simulink model "ZT_VehCtrl_18B"  (R2018b)
settings: Solver=FixedStepAuto  StartTime=0.0  StopTime=inf  FixedStep=0.005  RelTol=1e-3
InitFcn:
  | mbd_mpc_consistency_checks(bdroot(gcs));
undefined symbols (not defined in the file): ANG_DEAD, BMS_NormalPwr, BrkPrsByBrkPct_TB_X, BrkPrsByBrkPct_TB_Y, DELAY_DISCHARGE, DELAY_RCUOFF, DRV_BACKWARD, DRV_BRAKE, DRV_FORWARD, DRV_NEUTRAL, DRV_PARK, DRV_UNPARK, DRV_ZEROTURN, EPB_LOCK, EPB_UNLOCK, ExtraLoadPwr, FanOff, fifo_0_vect, fifo_1_vect, HiFanReq, HV_finished, HV_No_Active, HV_POWER_OFF, HV_POWER_ON, HVDown, HVON, KaTLS_v_DrgUp_X_VehSpd, KeFTM_s_Way1OffDlyTime, KeFTM_TK_Way1CoolLv2OffBatTemp, KeFTM_TK_Way1CoolLv2OffMtrTemp, KeFTM_TK_Way1CoolLv2OnBatTemp, KeFTM_TK_Way1CoolLv2OnMtrTemp, KeFTM_TK_Way1CoolLv3OffBatTemp, KeFTM_TK_Way1CoolLv3OffMtrTemp, KeFTM_TK_Way1CoolLv3OnBatTemp, KeFTM_TK_Way1CoolLv3OnMtrTemp, KeFTM_TK_Way1CoolLv4OffBatTemp, KeFTM_TK_Way1CoolLv4OffMtrTemp, KeFTM_TK_Way1CoolLv4OnBatTemp, KeFTM_TK_Way1CoolLv4OnMtrTemp, Kp1, Kp2, LowFanReq, LQFP, MtrPwrFactor_RCU, MtrPwrHighToMidThd, MtrPwrLowToMidThd, MtrPwrMidToHighThd, MtrPwrMidToLowThd, MtrTrqMax, PCT_DEAD, Precharge, PTO_1000, PTO_540, pts1_fifo_0_vect, pts1_fifo_1_vect, pts2_fifo_0_vect, pts2_fifo_1_vect, pts3_fifo_0_vect, pts3_fifo_1_vect ... (+24)
libraries: mbd_mpc574x_ec_toolbox x124, canmsglib x72, simulink x57
(part 2 of 11)

== system ZT_VehCtrl_18B/Initialization & SPI timer1 ==
  note: 由于SPI0用了两个片选，SPI3只用了一个片选（没算EEPROM）。
      | 因此直接用方波就可以了。
      | 如果增加SPI控制，建议使用StateFlow构造激活函数。
      | 由于模版使用的0.01s的仿真步长，这里构造周期为0.02s,占空比为0.5的方波。
  note: SPI3
  note: SPI0
  CS1 LS : Subsystem
  CS2 CANB : Subsystem
  CS3 LS : Subsystem
  CS5 LS : Subsystem
  Chart : Stateflow chart  TreatAsAtomicUnit=on
  Chart1 : Stateflow chart  TreatAsAtomicUnit=on
  Chart2 : Stateflow chart  TreatAsAtomicUnit=on
  Compare To Constant : simulink/Logic and Bit Operations/Compare To Constant  relop===  const=9  OutDataTypeStr=boolean
  Compare To Constant1 : simulink/Logic and Bit Operations/Compare To Constant  relop===  const=9  OutDataTypeStr=boolean
  Constant : Constant
  Data Store Read : DataStoreRead  DataStoreName=VCU_Mode
  Data Store Read1 : DataStoreRead  DataStoreName=ResetFlg
  Data Store Read2 : DataStoreRead  DataStoreName=Init_flg_SPI
  Data Store Write : DataStoreWrite  DataStoreName=VCU_Mode
  Data Store Write2 : DataStoreWrite  DataStoreName=SPI0_CS
  Data Store Write3 : DataStoreWrite  DataStoreName=SPI3_CS
  Data Store Write4 : DataStoreWrite  DataStoreName=Init_flg_SPI
  Data Type Conversion{,1..3} (4 alike) : DataTypeConversion
  If : If  IfExpression=u1 == 1  ShowElse=off
  If1 : If  IfExpression=u1 == 1  ShowElse=off
  If2 : If  IfExpression=u1 == 2  ShowElse=off
  If3 : If  IfExpression=u1 == 2  ShowElse=off
  Logical Operator : Logic  AllPortsSameDT=off  OutDataTypeStr=boolean
  Pulse Generator : DiscretePulseGenerator  PulseType=Time based  Period=0.01  PulseWidth=50
  wires:
  If/1 -> CS2 CANB/Action
  Chart/1(Flg) -> Data Type Conversion3/1
  Data Store Read2/1 -> Chart/2(InitFlg)
  If1/1 -> CS1 LS/Action
  Chart2/1(Flg) -> If3/1, [SPI3_flg], If/1
  Data Store Read/1 -> Chart2/1(VcuMode), Chart1/1(VcuMode)
  If2/1 -> CS5 LS/Action
  [SPI0_flg] -> Compare To Constant/1
  [SPI3_flg] -> Compare To Constant1/1
  Compare To Constant/1 -> Logical Operator/1
  Compare To Constant1/1 -> Logical Operator/2
  Logical Operator/1 -> Data Type Conversion2/1
  If3/1 -> CS3 LS/Action
  Pulse Generator/1 -> Data Type Conversion/1
  Constant/1 -> Data Type Conversion1/1
  Data Type Conversion/1 -> Data Store Write2/1
  Data Type Conversion1/1 -> Data Store Write3/1
  Data Type Conversion2/1 -> Data Store Write4/1
  Data Type Conversion3/1 -> Data Store Write/1
  Chart1/1(Flg) -> If1/1, [SPI0_flg], If2/1
  Data Store Read1/1 -> Chart/1(ResetFlg)

== system ZT_VehCtrl_18B/Power Managment ==
  PowerMode : Inport
  Data Type Conversion : DataTypeConversion
  HS1 : mbd_mpc574x_ec_toolbox/GPIO Blocks/Digital_Output  Priority=1  gpio_pin=PTF6: [SIUL2_GPIO86 | General Purpose IO PF[6]]  gpio_drive_strength=Disabled
  HS4 : mbd_mpc574x_ec_toolbox/GPIO Blocks/Digital_Output  Priority=1  gpio_pin=PTA13: [SIUL2_GPIO13 | General Purpose IO PA[13]]  gpio_drive_strength=Disabled
  wires:
  PowerMode/1 -> Data Type Conversion/1
  Data Type Conversion/1 -> HS4/1, HS1/1

== system ZT_VehCtrl_18B/SPI_EEPROM ==
  Data Store Memory : DataStoreMemory  DataStoreName=A_write  ReadBeforeWriteMsg=warning  WriteAfterWriteMsg=warning  WriteAfterReadMsg=warning  ShowAdditionalParam=off  OutDataTypeStr=single
      settings: RTWStateStorageClass=ExportedGlobal
  Data Store Memory10 : DataStoreMemory  DataStoreName=A_read  ReadBeforeWriteMsg=warning  WriteAfterWriteMsg=warning  WriteAfterReadMsg=warning  ShowAdditionalParam=off  OutDataTypeStr=single
      settings: RTWStateStorageClass=ExportedGlobal
  Data Store Memory18 : DataStoreMemory  DataStoreName=SPI0_CTRL0  ReadBeforeWriteMsg=warning  WriteAfterWriteMsg=warning  WriteAfterReadMsg=warning  ShowAdditionalParam=off  OutDataTypeStr=uint8
      settings: RTWStateStorageClass=ExportedGlobal
  Data Store Read : DataStoreRead  DataStoreName=SPI0_CTRL0
  SPI_read : Subsystem  TreatAsAtomicUnit=on
  SPI_write : Subsystem  TreatAsAtomicUnit=on
  Switch Case : SwitchCase  CaseConditions={1,2}  ShowDefaultCase=off
  wires:
  Data Store Read/1 -> Switch Case/1
  Switch Case/2 -> SPI_write/Action
  Switch Case/1 -> SPI_read/Action

== system ZT_VehCtrl_18B/SigIn ==
  note: CAN0
  note: HardWareSignalIn
  note: CAN1
  AI : Subsystem
  "CAN0 " : Subsystem  TreatAsAtomicUnit=on
      settings: RTWSystemCode=Nonreusable function
  CAN0_Rx_500 : mbd_mpc574x_ec_toolbox/Communication Blocks/CAN Blocks/FCAN_Isr  can_instance=0  can_event=Rx Complete
      settings: SourceProductName=NXP Model-Based Design Toolbox for MPC57xx MCUs
  CAN1 : Subsystem  TreatAsAtomicUnit=on
      settings: RTWSystemCode=Nonreusable function
  CAN1_Rx_500 : mbd_mpc574x_ec_toolbox/Communication Blocks/CAN Blocks/FCAN_Isr  can_instance=1  can_event=Rx Complete
      settings: SourceProductName=NXP Model-Based Design Toolbox for MPC57xx MCUs
  DI : Subsystem
  PWM : Subsystem
  Terminator{,3..5,8} (5 alike) : Terminator
  MCU_FL : Outport  VectorParamsAs1DForOutWhenUnconnected=on
  MCU_FR : Outport  Port=2  VectorParamsAs1DForOutWhenUnconnected=on
  MCU_RL : Outport  Port=3  VectorParamsAs1DForOutWhenUnconnected=on
  MCU_RR : Outport  Port=4  VectorParamsAs1DForOutWhenUnconnected=on
  MCU1 : Outport  Port=5  VectorParamsAs1DForOutWhenUnconnected=on
  MCU2 : Outport  Port=6  VectorParamsAs1DForOutWhenUnconnected=on
  HVC : Outport  Port=7  VectorParamsAs1DForOutWhenUnconnected=on
  ACU : Outport  Port=8  VectorParamsAs1DForOutWhenUnconnected=on
  PDU : Outport  Port=9  VectorParamsAs1DForOutWhenUnconnected=on
  TWV : Outport  Port=10  VectorParamsAs1DForOutWhenUnconnected=on
  TMS : Outport  Port=11  VectorParamsAs1DForOutWhenUnconnected=on
  ISG : Outport  Port=12  VectorParamsAs1DForOutWhenUnconnected=on
  wires:
  CAN1_Rx_500/2 -> Terminator4/1
  CAN1_Rx_500/6 -> CAN1/4(timestamp)
  CAN1_Rx_500/4 -> CAN1/2(Data)
  CAN1_Rx_500/3 -> CAN1/1(ID)
  CAN1_Rx_500/5 -> CAN1/3(length)
  CAN0_Rx_500/5 -> "CAN0 "/3(length)
  CAN0_Rx_500/3 -> "CAN0 "/1(ID)
  CAN0_Rx_500/4 -> "CAN0 "/2(Data)
  CAN0_Rx_500/6 -> "CAN0 "/4(timestamp)
  CAN0_Rx_500/1 -> "CAN0 "/Trigger
  CAN0_Rx_500/2 -> Terminator8/1
  "CAN0 "/1(BMS) -> MCU_FL/1
  "CAN0 "/2(OBC) -> MCU_FR/1
  "CAN0 "/4("BRS ") -> MCU_RR/1
  "CAN0 "/3(TMS) -> MCU_RL/1
  CAN1_Rx_500/1 -> CAN1/Trigger
  PWM/1(PWMIn) -> Terminator/1
  DI/1(DI) -> Terminator3/1
  AI/1(AI) -> Terminator5/1
  CAN1/1(MCU1) -> MCU1/1
  CAN1/3(HVC) -> HVC/1
  CAN1/7(TMS) -> TMS/1
  CAN1/8("ISG ") -> ISG/1
  CAN1/6(TWV) -> TWV/1
  CAN1/5(PDU) -> PDU/1
  CAN1/4(ACU) -> ACU/1
  CAN1/2(MCU2) -> MCU2/1

== system ZT_VehCtrl_18B/SigOut ==
  note: 10ms
  note: 500ms
  note: 100ms
  note: 200ms
  BMS_OUT : Inport
  ICU : Inport  Port=2
  TMS_OUT1 : Inport  Port=3
  BRS_OUT : Inport  Port=4
  "DCDC_OUT " : Inport  Port=5
  HVC_OUT : Inport  Port=6
  MCU_OUT : Inport  Port=7
  ACU_OUT : Inport  Port=8
  PDU_OUT : Inport  Port=9
  TM_OUT : Inport  Port=10
  ISG_OUT : Inport  Port=11
  TWV_OUT : Inport  Port=12
  ACU : Subsystem  TreatAsAtomicUnit=on  SystemSampleTime=0.01
  BMS : Subsystem  TreatAsAtomicUnit=on  SystemSampleTime=0.01
  BRS : Subsystem  TreatAsAtomicUnit=on  SystemSampleTime=0.01
  DCDC : Subsystem  TreatAsAtomicUnit=on  SystemSampleTime=0.01
  "GPIO " : Subsystem
  HVC : Subsystem  TreatAsAtomicUnit=on  SystemSampleTime=0.01
  "ICU1 " : Subsystem  TreatAsAtomicUnit=on  SystemSampleTime=0.01
  ICU2 : Subsystem  TreatAsAtomicUnit=on  SystemSampleTime=0.01
  ISG : Subsystem  TreatAsAtomicUnit=on  SystemSampleTime=0.01
  MCU : Subsystem  TreatAsAtomicUnit=on  SystemSampleTime=0.01
  PDU : Subsystem  TreatAsAtomicUnit=on  SystemSampleTime=0.01
  Pulse Generator : DiscretePulseGenerator  PulseType=Time based  Period=0.1  PulseWidth=50
  Pulse Generator1 : DiscretePulseGenerator  PulseType=Time based  Period=0.01  PulseWidth=50
  Pulse Generator2 : DiscretePulseGenerator  PulseType=Time based  Period=0.5  PulseWidth=50
  Pulse Generator6 : DiscretePulseGenerator  PulseType=Time based  Period=0.2  PulseWidth=50
  Rate Transition{,1..4,6..13} (13 alike) : RateTransition
  TM : Subsystem  TreatAsAtomicUnit=on  SystemSampleTime=0.01
  TMS1 : Subsystem  TreatAsAtomicUnit=on  SystemSampleTime=0.01
  TWV : Subsystem  TreatAsAtomicUnit=on  SystemSampleTime=0.01
  wires:
  Pulse Generator2/1 -> ICU2/Trigger
  BMS_OUT/1 -> Rate Transition/1
  Rate Transition/1 -> BMS/1("BMS_OUT ")
  Rate Transition4/1 -> ICU2/1("ICU_OUT ")
  Pulse Generator/1 -> BRS/Trigger, "ICU1 "/Trigger, DCDC/Trigger, HVC/Trigger, TWV/Trigger, PDU/Trigger, ACU/Trigger, BMS/Trigger
  ICU/1 -> Rate Transition4/1, Rate Transition6/1
  Rate Transition6/1 -> "ICU1 "/1("ICU_OUT ")
  TMS_OUT1/1 -> Rate Transition7/1
  Rate Transition7/1 -> TMS1/1("TMS_OUT ")
  Pulse Generator6/1 -> TMS1/Trigger
  BRS_OUT/1 -> Rate Transition8/1
  Rate Transition8/1 -> BRS/1("BRS_OUT ")
  Rate Transition1/1 -> DCDC/1("DCDC_OUT ")
  "DCDC_OUT "/1 -> Rate Transition1/1
  HVC_OUT/1 -> Rate Transition2/1
  Rate Transition2/1 -> HVC/1("HVC_OUT ")
  Rate Transition3/1 -> MCU/1("MCU_OUT ")
  MCU_OUT/1 -> Rate Transition3/1
  Rate Transition9/1 -> ACU/1("ACU_OUT ")
  ACU_OUT/1 -> Rate Transition9/1
  PDU_OUT/1 -> Rate Transition10/1
  Rate Transition10/1 -> PDU/1("PDU_OUT ")
  TM_OUT/1 -> Rate Transition11/1
  Rate Transition11/1 -> TM/1("TM_OUT ")
  Rate Transition12/1 -> ISG/1("ISG_OUT ")
  ISG_OUT/1 -> Rate Transition12/1
  Pulse Generator1/1 -> MCU/Trigger, ISG/Trigger, TM/Trigger
  Rate Transition13/1 -> TWV/1("TWV_OUT ")
  TWV_OUT/1 -> Rate Transition13/1

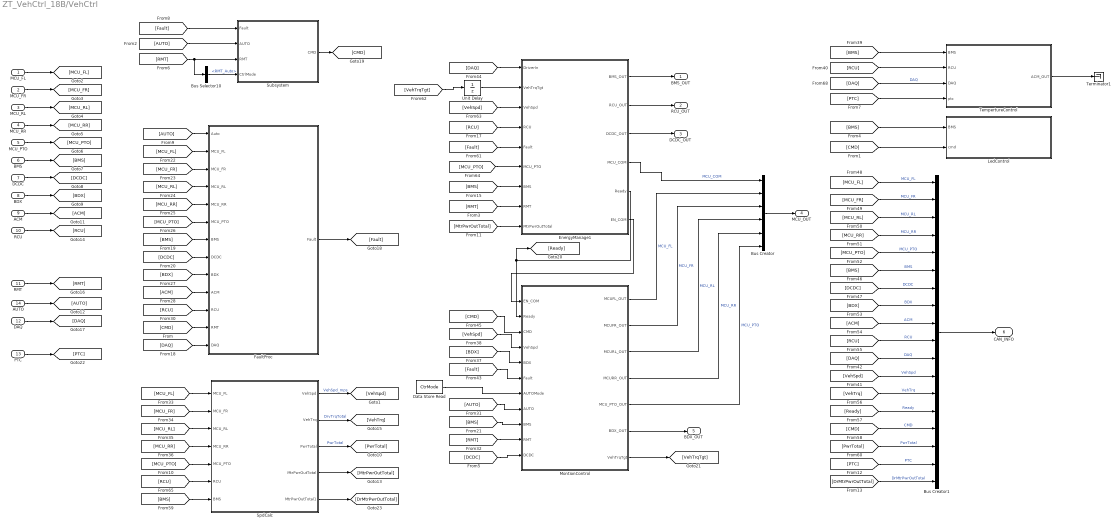
== system ZT_VehCtrl_18B/VehCtrl ==
  MCU_FL : Inport
  MCU_FR : Inport  Port=2
  MCU_RL : Inport  Port=3
  MCU_RR : Inport  Port=4
  MCU_PTO : Inport  Port=5
  BMS : Inport  Port=6
  DCDC : Inport  Port=7
  BDX : Inport  Port=8
  ACM : Inport  Port=9
  RCU : Inport  Port=10
  RMT : Inport  Port=11
  DAQ : Inport  Port=12
  "PTC " : Inport  Port=13
  AUTO : Inport  Port=14
  Bus Creator : BusCreator  Inputs=6
  Bus Creator1 : BusCreator  Inputs=18
  Bus Selector10 : BusSelector  OutputSignals=RMT3.RMT_Auto
  Data Store Read : DataStoreRead  DataStoreName=CtrMode
  EnergyManage1 : Subsystem
  FaultProc : Subsystem
  LedControl : Subsystem
  MontionControl : Subsystem
  SpdCalc : Subsystem
  Subsystem : Subsystem
  TempertureControl : Subsystem
  Terminator1 : Terminator
  Unit Delay : UnitDelay  SampleTime=-1
  BMS_OUT : Outport
  RCU_OUT : Outport  Port=2
  DCDC_OUT : Outport  Port=3
  MCU_OUT : Outport  Port=4
  BDX_OUT : Outport  Port=5
  CAN_INFO : Outport  Port=6
  wires:
  MCU_FL/1 -> [MCU_FL]
  MCU_FR/1 -> [MCU_FR]
  MCU_RR/1 -> [MCU_RR]
  MCU_RL/1 -> [MCU_RL]
  DCDC/1 -> [DCDC]
  BDX/1 -> [BDX]
  BMS/1 -> [BMS]
  MCU_PTO/1 -> [MCU_PTO]
  RMT/1 -> [RMT]
  DAQ/1 -> [DAQ]
  RCU/1 -> [RCU]
  ACM/1 -> [ACM]
  [RCU] -> EnergyManage1/4(RCU)
  [MCU_FL] -> FaultProc/2(MCU_FL)
  [MCU_FR] -> FaultProc/3(MCU_FR)
  [MCU_RL] -> FaultProc/4(MCU_RL)
  [MCU_RR] -> FaultProc/5(MCU_RR)
  [MCU_PTO] -> FaultProc/6(MCU_PTO)
  [BMS] -> FaultProc/7(BMS)
  [DCDC] -> FaultProc/8(DCDC)
  [BDX] -> FaultProc/9(BDX)
  [ACM] -> FaultProc/10(ACM)
  [RCU] -> FaultProc/11(RCU)
  [CMD] -> FaultProc/12(RMT)
  [DAQ] -> FaultProc/13(DAQ)
  [BDX] -> MontionControl/5(BDX)
  [VehSpd] -> MontionControl/4(VehSpd)
  FaultProc/1(Fault) -> [Fault]
  [Fault] -> MontionControl/6(Fault)
  [DAQ] -> EnergyManage1/1(DriverIn)
  [CMD] -> MontionControl/3(CMD)
  [Fault] -> EnergyManage1/5(Fault)
  MontionControl/7(VehTrqTgt) -> [VehTrqTgt]
  [VehTrqTgt] -> Unit Delay/1
  [VehSpd] -> EnergyManage1/3(VehSpd)
  [MCU_PTO] -> EnergyManage1/6(MCU_PTO)
  [BMS] -> EnergyManage1/7(BMS)
  Unit Delay/1 -> EnergyManage1/2(VehTrqTgt)
  EnergyManage1/4(MCU_COM) -> Bus Creator/1  "MCU_COM"
  Bus Creator/1 -> MCU_OUT/1
  EnergyManage1/1(BMS_OUT) -> BMS_OUT/1
  EnergyManage1/2(RCU_OUT) -> RCU_OUT/1
  EnergyManage1/3(DCDC_OUT) -> DCDC_OUT/1
  MontionControl/1(MCUFL_OUT) -> Bus Creator/2  "MCU_FL"
  MontionControl/2(MCUFR_OUT) -> Bus Creator/3  "MCU_FR"
  MontionControl/3(MCURL_OUT) -> Bus Creator/4  "MCU_RL"
  MontionControl/4(MCURR_OUT) -> Bus Creator/5  "MCU_RR"
  MontionControl/5(MCU_PTO_OUT) -> Bus Creator/6  "MCU_PTO"
  MontionControl/6(BDX_OUT) -> BDX_OUT/1
  "PTC "/1 -> [PTC]
  AUTO/1 -> [AUTO]
  [AUTO] -> Subsystem/2(AUTO)
  Subsystem/1(CMD) -> [CMD]
  Data Store Read/1 -> MontionControl/7(AUTOMode)
  [AUTO] -> MontionControl/8(AUTO)
  Bus Selector10/1 -> Subsystem/4(CtrlMode)  "<RMT_Auto>"
  [RMT] -> Subsystem/3(RMT), Bus Selector10/1
  [RMT] -> EnergyManage1/8("RMT ")
  [CMD] -> LedControl/2(cmd)
  TempertureControl/1(ACM_OUT) -> Terminator1/1
  [RCU] -> TempertureControl/2(RCU)
  [BMS] -> TempertureControl/1(BMS)
  [BMS] -> MontionControl/9(BMS)
  [RMT] -> MontionControl/10(RMT)
  [DAQ] -> TempertureControl/3(DAQ)  "DAQ"
  [BMS] -> LedControl/1(BMS)
  [DCDC] -> MontionControl/11(DCDC)
  [PTC] -> TempertureControl/4(ptc)
  [Fault] -> Subsystem/1(Fault)
  [AUTO] -> FaultProc/1(Auto)
  [MCU_RR] -> SpdCalc/4(MCU_RR)
  [MCU_FR] -> SpdCalc/2(MCU_FR)
  [MCU_FL] -> SpdCalc/1(MCU_FL)
  [MCU_PTO] -> SpdCalc/5(MCU_PTO)
  [BMS] -> SpdCalc/7(BMS)
  SpdCalc/2("VehTrq ") -> [VehTrq]  "DrvTrqTotal"
  [RCU] -> SpdCalc/6(RCU)
  SpdCalc/5(MtrPwrOutTotal1) -> [DrMtrPwrOutTotal]
  SpdCalc/4(MtrPwrOutTotal) -> [MtrPwrOutTotal]
  SpdCalc/1(VehSpd) -> [VehSpd]  "VehSpd_mps"
  SpdCalc/3(PwrTotal) -> [PwrTotal]  "PwrTotal"
  [MCU_RL] -> SpdCalc/3(MCU_RL)
  EnergyManage1/6(EN_COM) -> MontionControl/1(EN_COM)
  EnergyManage1/5(Ready) -> MontionControl/2(Ready), [Ready]
  [MtrPwrOutTotal] -> EnergyManage1/9(MtrPwrOutTotal)
  Bus Creator1/1 -> CAN_INFO/1
  [BMS] -> Bus Creator1/6  "BMS"
  [MCU_FR] -> Bus Creator1/2  "MCU_FR"
  [PwrTotal] -> Bus Creator1/16  "PwrTotal"
  [MCU_RL] -> Bus Creator1/3  "MCU_RL"
  [DAQ] -> Bus Creator1/11  "DAQ"
  [BDX] -> Bus Creator1/8  "BDX"
  [MCU_RR] -> Bus Creator1/4  "MCU_RR"
  [VehSpd] -> Bus Creator1/12  "VehSpd"
  [CMD] -> Bus Creator1/15  "CMD"
  [DrMtrPwrOutTotal] -> Bus Creator1/18  "DrMtrPwrOutTotal"
  [ACM] -> Bus Creator1/9  "ACM"
  [Ready] -> Bus Creator1/14  "Ready"
  [MCU_PTO] -> Bus Creator1/5  "MCU_PTO"
  [PTC] -> Bus Creator1/17  "PTC"
  [DCDC] -> Bus Creator1/7  "DCDC"
  [MCU_FL] -> Bus Creator1/1  "MCU_FL"
  [VehTrq] -> Bus Creator1/13  "VehTrq"
  [RCU] -> Bus Creator1/10  "RCU"

== system ZT_VehCtrl_18B/Initialization & SPI timer1/CS1 LS ==
  Action Port : ActionPort  ActionType=then
  Chart : Stateflow chart  TreatAsAtomicUnit=on
  Data Type Conversion{,1,3..4} (4 alike) : DataTypeConversion
  Demux1 : Demux  Outputs=2
  SPI_Master_Transfer_To1 : mbd_mpc574x_ec_toolbox/Communication Blocks/SPI Blocks/SPI_Master_Transfer  Priority=2  InstanceNumber=0  xfermode=Non blocking  timeout=50  spi_upd=on  WhichPCS=5
  Subsystem : Subsystem  Commented=on
  Terminator : Terminator
  Terminator1 : Terminator
  Vector Concatenate1 : Concatenate
  wires:
  SPI_Master_Transfer_To1/1 -> Demux1/1
  Data Type Conversion3/1 -> Terminator/1
  Vector Concatenate1/1 -> SPI_Master_Transfer_To1/1
  Demux1/2 -> Data Type Conversion4/1
  Data Type Conversion4/1 -> Terminator1/1
  Demux1/1 -> Data Type Conversion3/1
  Chart/1(high) -> Data Type Conversion/1
  Chart/2(low) -> Data Type Conversion1/1
  Data Type Conversion/1 -> Vector Concatenate1/1
  Data Type Conversion1/1 -> Vector Concatenate1/2

== system ZT_VehCtrl_18B/Initialization & SPI timer1/CS2 CANB ==
  Action Port : ActionPort  ActionType=then
  Constant : Constant  Value=2
  Constant1 : Constant  Value=7
  Data Type Conversion : DataTypeConversion  OutDataTypeStr=uint8
  Data Type Conversion1 : DataTypeConversion  OutDataTypeStr=uint8
  Data Type Conversion2 : DataTypeConversion
  Data Type Conversion3 : DataTypeConversion
  Demux2 : Demux  Outputs=2
  SPI_Master_Transfer_To2 : mbd_mpc574x_ec_toolbox/Communication Blocks/SPI Blocks/SPI_Master_Transfer  Priority=2  InstanceNumber=3  xfermode=Non blocking  timeout=50  spi_upd=on  WhichPCS=2
  Terminator : Terminator
  Terminator1 : Terminator
  Vector Concatenate2 : Concatenate
  wires:
  Vector Concatenate2/1 -> SPI_Master_Transfer_To2/1
  Demux2/2 -> Data Type Conversion1/1
  Data Type Conversion2/1 -> Vector Concatenate2/2
  SPI_Master_Transfer_To2/1 -> Demux2/1
  Data Type Conversion1/1 -> Terminator1/1
  Data Type Conversion/1 -> Terminator/1
  Demux2/1 -> Data Type Conversion/1
  Data Type Conversion3/1 -> Vector Concatenate2/1
  Constant/1 -> Data Type Conversion3/1
  Constant1/1 -> Data Type Conversion2/1

== system ZT_VehCtrl_18B/Initialization & SPI timer1/CS3 LS ==
  note: 80-0101 0000 - 对A组端口控制模式进行设置
      | 96-0110 0000 - 对B组端口控制模式进行设置
      | 40-0010 1100 -使用SPI控制端口
      |
      | 其中端口1,2,5,6即为复用PWM端口，这里设置为引脚控制（A组），其余端口设置为SPI控制
  Action Port : ActionPort  ActionType=then
  Chart : Stateflow chart  TreatAsAtomicUnit=on
  Data Type Conversion : DataTypeConversion  OutDataTypeStr=uint8
  Data Type Conversion1 : DataTypeConversion  OutDataTypeStr=uint8
  Data Type Conversion2 : DataTypeConversion
  Data Type Conversion3 : DataTypeConversion
  Demux2 : Demux  Outputs=2
  Manual Switch : ManualSwitch  CurrentSetting=0
  PIN : Constant  Value=2
  SPI : Constant  Value=0
  SPI_Master_Transfer_To2 : mbd_mpc574x_ec_toolbox/Communication Blocks/SPI Blocks/SPI_Master_Transfer  Priority=2  InstanceNumber=3  xfermode=Non blocking  timeout=50  spi_upd=on  WhichPCS=3
  Subsystem : Subsystem  Commented=on
  Terminator2 : Terminator
  Terminator3 : Terminator
  Vector Concatenate1 : Concatenate
  wires:
  Data Type Conversion1/1 -> Terminator3/1
  Data Type Conversion/1 -> Terminator2/1
  Demux2/1 -> Data Type Conversion/1
  SPI_Master_Transfer_To2/1 -> Demux2/1
  Demux2/2 -> Data Type Conversion1/1
  Chart/2(low) -> Data Type Conversion3/1
  Vector Concatenate1/1 -> SPI_Master_Transfer_To2/1
  Data Type Conversion2/1 -> Vector Concatenate1/1
  Data Type Conversion3/1 -> Vector Concatenate1/2
  Chart/1(high) -> Data Type Conversion2/1
  PIN/1 -> Manual Switch/2
  SPI/1 -> Manual Switch/1
  Manual Switch/1 -> [Mode]
  [Mode] -> Chart/1(mode)

== system ZT_VehCtrl_18B/Initialization & SPI timer1/CS5 LS ==
  Action Port : ActionPort  ActionType=then
  Chart : Stateflow chart  TreatAsAtomicUnit=on
  Data Type Conversion{,1,3..4} (4 alike) : DataTypeConversion
  Demux1 : Demux  Outputs=2
  SPI_Master_Transfer_To1 : mbd_mpc574x_ec_toolbox/Communication Blocks/SPI Blocks/SPI_Master_Transfer  Priority=2  InstanceNumber=0  xfermode=Non blocking  timeout=50  spi_upd=on  WhichPCS=1
  Subsystem : Subsystem  Commented=on
  Terminator : Terminator
  Terminator1 : Terminator
  Vector Concatenate1 : Concatenate
  wires:
  SPI_Master_Transfer_To1/1 -> Demux1/1
  Demux1/1 -> Data Type Conversion3/1
  Data Type Conversion3/1 -> Terminator/1
  Demux1/2 -> Data Type Conversion4/1
  Data Type Conversion4/1 -> Terminator1/1
  Chart/2(low) -> Data Type Conversion1/1
  Vector Concatenate1/1 -> SPI_Master_Transfer_To1/1
  Data Type Conversion/1 -> Vector Concatenate1/1
  Data Type Conversion1/1 -> Vector Concatenate1/2
  Chart/1(high) -> Data Type Conversion/1

== system ZT_VehCtrl_18B/SPI_EEPROM/SPI_read ==
  Action Port : ActionPort
  "Address_High " : Constant  Value=hex2dec('FF')  OutDataTypeStr=uint8
  Address_Low : Constant  Value=hex2dec('FF')
  Bitwise AND : simulink/Logic and Bit Operations/Bitwise Operator  logicop=AND  UseBitMask=on  BitMask=hex2dec('00FF')  BitMaskRealWorld=Stored Integer
  Constant : Constant  Value=0
  Data Store Write : DataStoreWrite  DataStoreName=A_read
  Data Type Conversion{,1,3..8} (8 alike) : DataTypeConversion  OutDataTypeStr=uint8
  Data Type Conversion2 : DataTypeConversion
  Demux1 : Demux
  SPI_Master_Transfer_To1 : mbd_mpc574x_ec_toolbox/Communication Blocks/SPI Blocks/SPI_Master_Transfer  Priority=2  InstanceNumber=0  xfermode=Non blocking  timeout=50  spi_upd=on  WhichPCS=0
  Terminator : Terminator
  Terminator1 : Terminator
  Terminator2 : Terminator
  Vector Concatenate1 : Concatenate  NumInputs=4
  read_set : Constant  Value=3  OutDataTypeStr=uint8
  wires:
  "Address_High "/1 -> Data Type Conversion1/1
  read_set/1 -> Data Type Conversion/1
  Data Type Conversion1/1 -> Vector Concatenate1/2  "d1"
  Data Type Conversion/1 -> Vector Concatenate1/1  "d0"
  Address_Low/1 -> Data Type Conversion6/1
  Demux1/2 -> Data Type Conversion4/1
  Vector Concatenate1/1 -> SPI_Master_Transfer_To1/1
  Demux1/1 -> Data Type Conversion3/1
  SPI_Master_Transfer_To1/1 -> Demux1/1
  Data Type Conversion3/1 -> Terminator/1  "r0"
  Data Type Conversion8/1 -> Bitwise AND/1  "r3"
  Bitwise AND/1 -> Data Type Conversion2/1
  Data Type Conversion2/1 -> Data Store Write/1
  Constant/1 -> Data Type Conversion7/1
  Data Type Conversion6/1 -> Vector Concatenate1/3  "d2"
  Data Type Conversion7/1 -> Vector Concatenate1/4  "d3"
  Demux1/3 -> Data Type Conversion5/1
  Data Type Conversion4/1 -> Terminator1/1  "r1"
  Data Type Conversion5/1 -> Terminator2/1  "r2"
  Demux1/4 -> Data Type Conversion8/1

== system ZT_VehCtrl_18B/SPI_EEPROM/SPI_write ==
  Action Port : ActionPort
  Data Store Memory : DataStoreMemory  DataStoreName=Write_Ctrl  ReadBeforeWriteMsg=warning  WriteAfterWriteMsg=warning  WriteAfterReadMsg=warning  InitialValue=1  ShowAdditionalParam=off  OutDataTypeStr=uint8
      settings: RTWStateStorageClass=ExportedGlobal
  Data Store Read : DataStoreRead  DataStoreName=Write_Ctrl
  SPI_enable : Subsystem  TreatAsAtomicUnit=on
  SPI_write : Subsystem  TreatAsAtomicUnit=on
  Switch Case : SwitchCase  CaseConditions={1,2}  ShowDefaultCase=off
  wires:
  Data Store Read/1 -> Switch Case/1
  Switch Case/2 -> SPI_write/Action
  Switch Case/1 -> SPI_enable/Action

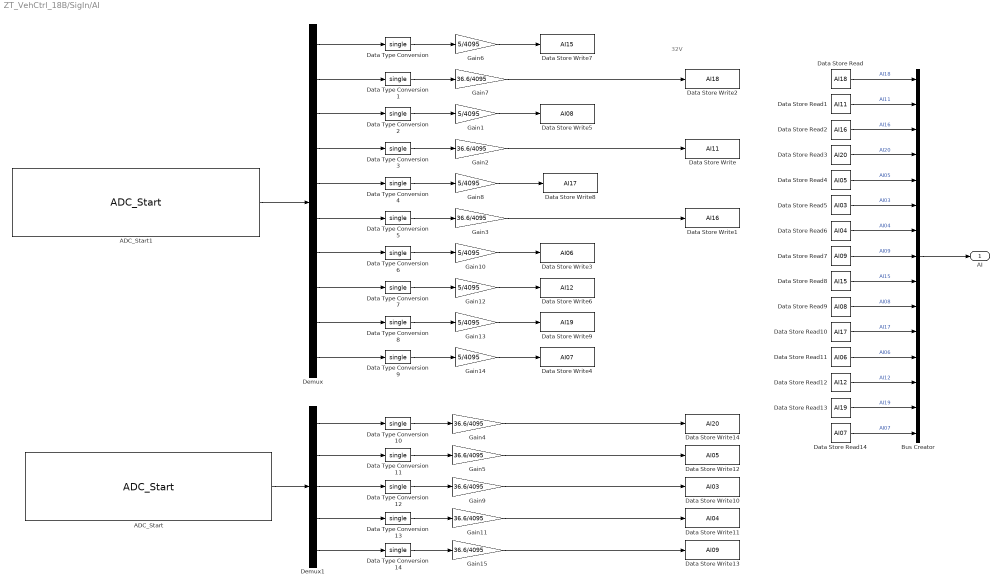
== system ZT_VehCtrl_18B/SigIn/AI ==
  note: 32V
  ADC_Start : mbd_mpc574x_ec_toolbox/Motor Control Blocks/ADC Blocks/ADC_Start  adc_instance=1  interrupt=off  presample=off
  ADC_Start1 : mbd_mpc574x_ec_toolbox/Motor Control Blocks/ADC Blocks/ADC_Start  adc_instance=0  interrupt=off  presample=off
  Bus Creator : BusCreator  Inputs=15
  Data Store Read : DataStoreRead  DataStoreName=AI18
  Data Store Read1 : DataStoreRead  DataStoreName=AI11
  Data Store Read10 : DataStoreRead  DataStoreName=AI17
  Data Store Read11 : DataStoreRead  DataStoreName=AI06
  Data Store Read12 : DataStoreRead  DataStoreName=AI12
  Data Store Read13 : DataStoreRead  DataStoreName=AI19
  Data Store Read14 : DataStoreRead  DataStoreName=AI07
  Data Store Read2 : DataStoreRead  DataStoreName=AI16
  Data Store Read3 : DataStoreRead  DataStoreName=AI20
  Data Store Read4 : DataStoreRead  DataStoreName=AI05
  Data Store Read5 : DataStoreRead  DataStoreName=AI03
  Data Store Read6 : DataStoreRead  DataStoreName=AI04
  Data Store Read7 : DataStoreRead  DataStoreName=AI09
  Data Store Read8 : DataStoreRead  DataStoreName=AI15
  Data Store Read9 : DataStoreRead  DataStoreName=AI08
  Data Store Write : DataStoreWrite  DataStoreName=AI11
  Data Store Write1 : DataStoreWrite  DataStoreName=AI16
  Data Store Write10 : DataStoreWrite  DataStoreName=AI03
  Data Store Write11 : DataStoreWrite  DataStoreName=AI04
  Data Store Write12 : DataStoreWrite  DataStoreName=AI05
  Data Store Write13 : DataStoreWrite  DataStoreName=AI09
  Data Store Write14 : DataStoreWrite  DataStoreName=AI20
  Data Store Write2 : DataStoreWrite  DataStoreName=AI18
  Data Store Write3 : DataStoreWrite  DataStoreName=AI06
  Data Store Write4 : DataStoreWrite  DataStoreName=AI07
  Data Store Write5 : DataStoreWrite  DataStoreName=AI08
  Data Store Write6 : DataStoreWrite  DataStoreName=AI12
  Data Store Write7 : DataStoreWrite  DataStoreName=AI15
  Data Store Write8 : DataStoreWrite  DataStoreName=AI17
  Data Store Write9 : DataStoreWrite  DataStoreName=AI19
  Data Type Conversion{,1..14} (15 alike) : DataTypeConversion  OutDataTypeStr=single
  Demux : Demux  Outputs=10
  Demux1 : Demux  Outputs=5
  Gain{1,6,8,10,12..14} (7 alike) : Gain  Gain=5/4095
  Gain{2..5,7,9,11,15} (8 alike) : Gain  Gain=36.6/4095  OutDataTypeStr=single
  AI : Outport
  wires:
  Demux/4 -> Data Type Conversion3/1
  ADC_Start1/1 -> Demux/1
  Demux/7 -> Data Type Conversion6/1
  Demux1/4 -> Data Type Conversion13/1
  Demux1/3 -> Data Type Conversion12/1
  ADC_Start/1 -> Demux1/1
  Demux1/2 -> Data Type Conversion11/1
  Demux1/5 -> Data Type Conversion14/1
  Demux1/1 -> Data Type Conversion10/1
  Demux/1 -> Data Type Conversion/1
  Demux/3 -> Data Type Conversion2/1
  Demux/2 -> Data Type Conversion1/1
  Demux/5 -> Data Type Conversion4/1
  Demux/8 -> Data Type Conversion7/1
  Demux/9 -> Data Type Conversion8/1
  Demux/10 -> Data Type Conversion9/1
  Demux/6 -> Data Type Conversion5/1
  Data Type Conversion/1 -> Gain6/1
  Gain6/1 -> Data Store Write7/1
  Data Type Conversion1/1 -> Gain7/1
  Data Type Conversion2/1 -> Gain1/1
  Data Type Conversion3/1 -> Gain2/1
  Data Type Conversion4/1 -> Gain8/1
  Data Type Conversion5/1 -> Gain3/1
  Data Type Conversion6/1 -> Gain10/1
  Data Type Conversion7/1 -> Gain12/1
  Data Type Conversion8/1 -> Gain13/1
  Data Type Conversion9/1 -> Gain14/1
  Data Type Conversion10/1 -> Gain4/1
  Data Type Conversion11/1 -> Gain5/1
  Data Type Conversion12/1 -> Gain9/1
  Data Type Conversion13/1 -> Gain11/1
  Data Type Conversion14/1 -> Gain15/1
  Gain7/1 -> Data Store Write2/1
  Gain1/1 -> Data Store Write5/1
  Gain2/1 -> Data Store Write/1
  Gain8/1 -> Data Store Write8/1
  Gain3/1 -> Data Store Write1/1
  Gain10/1 -> Data Store Write3/1
  Gain12/1 -> Data Store Write6/1
  Gain13/1 -> Data Store Write9/1
  Gain14/1 -> Data Store Write4/1
  Gain4/1 -> Data Store Write14/1
  Gain5/1 -> Data Store Write12/1
  Gain9/1 -> Data Store Write10/1
  Gain11/1 -> Data Store Write11/1
  Gain15/1 -> Data Store Write13/1
  Data Store Read/1 -> Bus Creator/1  "AI18"
  Data Store Read1/1 -> Bus Creator/2  "AI11"
  Data Store Read2/1 -> Bus Creator/3  "AI16"
  Data Store Read3/1 -> Bus Creator/4  "AI20"
  Data Store Read4/1 -> Bus Creator/5  "AI05"
  Data Store Read5/1 -> Bus Creator/6  "AI03"
  Data Store Read6/1 -> Bus Creator/7  "AI04"
  Data Store Read7/1 -> Bus Creator/8  "AI09"
  Data Store Read8/1 -> Bus Creator/9  "AI15"
  Data Store Read9/1 -> Bus Creator/10  "AI08"
  Data Store Read10/1 -> Bus Creator/11  "AI17"
  Data Store Read11/1 -> Bus Creator/12  "AI06"
  Data Store Read12/1 -> Bus Creator/13  "AI12"
  Data Store Read13/1 -> Bus Creator/14  "AI19"
  Data Store Read14/1 -> Bus Creator/15  "AI07"
  Bus Creator/1 -> AI/1

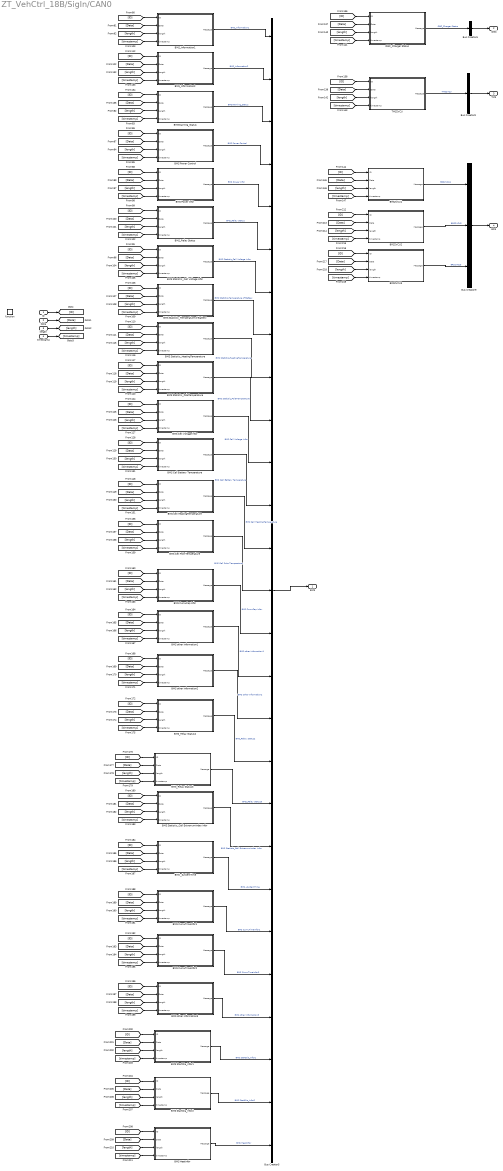
== system ZT_VehCtrl_18B/SigIn/CAN0  ==
  ID : Inport
  Data : Inport  Port=2
  length : Inport  Port=3
  timestamp : Inport  Port=4
  function : TriggerPort  TriggerType=function-call  VariantControl=Variant
  BMS Cell Battery Temperature : Subsystem
  BMS Cell HeatingTemperature : Subsystem
  BMS Cell Pole Temperature : Subsystem
  BMS Cell Voltage Infor : Subsystem
  BMS CumuCap Infor : Subsystem
  BMS CumuTimeInfor1 : Subsystem
  BMS CumuTimeInfor2 : Subsystem
  BMS HeatInfor : Subsystem
  BMS Power Control : Subsystem
  BMS Power Infor : Subsystem
  BMS StartDia_Infor1 : Subsystem
  BMS StartDia_Infor2 : Subsystem
  BMS Statistic_Cell ExtremumIndex Infor : Subsystem
  BMS Statistic_Cell Voltage Infor : Subsystem
  BMS Statistic_HeatingTemperature : Subsystem
  BMS Statistic_PoleTemperature : Subsystem
  BMS Statistic_Temperature of Battery : Subsystem
  "BMS _SystemTime " : Subsystem
  BMS other Information1 : Subsystem
  "BMS other Information2 " : Subsystem
  BMS other Information3 : Subsystem
  BMSWarning_Status : Subsystem
  BMS_Information1 : Subsystem
  BMS_Information2 : Subsystem
  BMS_Relay Status : Subsystem
  BMS_Relay Status2 : Subsystem
  BMS_Relay Status3 : Subsystem
  BRS2VCU1 : Subsystem
  BRS2VCU2 : Subsystem
  BRS2VCU3 : Subsystem
  Bus Creator5 : BusCreator  Inputs=27
  Bus Creator6 : BusCreator  Inputs=1
  Bus Creator8 : BusCreator  Inputs=1
  Bus Creator9 : BusCreator  Inputs=3
  OBC_Charger Status : Subsystem
  TMS2VCU : Subsystem
  BMS : Outport
  OBC : Outport  Port=2
  TMS : Outport  Port=3
  "BRS " : Outport  Port=4
  wires:
  [timestamp] -> BMS Statistic_Temperature of Battery/4(timestamp)
  [ID] -> BMS Cell Battery Temperature/1(ID)
  BMS Statistic_PoleTemperature/1(Message) -> Bus Creator5/10  "BMS Statistic_PoleTemperature"
  [Data] -> BMS_Relay Status/2(Data)
  BMS Statistic_Temperature of Battery/1(Message) -> Bus Creator5/8  "BMS Statistic_Temperature of Battery"
  BMS Statistic_HeatingTemperature/1(Message) -> Bus Creator5/9  "BMS Statistic_HeatingTemperature"
  [length] -> BMS Cell Battery Temperature/3(length)
  [timestamp] -> BMS Statistic_Cell Voltage Infor/4(timestamp)
  [length] -> BMS Statistic_Temperature of Battery/3(length)
  BMS Power Infor/1(Message) -> Bus Creator5/5  "BMS Power Infor"
  [timestamp] -> BMS Cell Battery Temperature/4(timestamp)
  [ID] -> BMS Statistic_PoleTemperature/1(ID)
  BMS Cell Battery Temperature/1(Message) -> Bus Creator5/12  "BMS Cell Battery Temperature"
  [Data] -> BMS Statistic_Cell Voltage Infor/2(Data)
  [length] -> BMS Statistic_PoleTemperature/3(length)
  [timestamp] -> BMS Statistic_PoleTemperature/4(timestamp)
  [Data] -> BMS Power Control/2(Data)
  [Data] -> BMS Statistic_PoleTemperature/2(Data)
  [Data] -> BMS Cell Voltage Infor/2(Data)
  BMS_Relay Status/1(Message) -> Bus Creator5/6  "BMS_Relay Status"
  [timestamp] -> BMSWarning_Status/4(timestamp)
  [ID] -> BMS Statistic_Cell Voltage Infor/1(ID)
  [Data] -> BMS Statistic_Temperature of Battery/2(Data)
  [length] -> BMSWarning_Status/3(length)
  [timestamp] -> BMS Statistic_HeatingTemperature/4(timestamp)
  Bus Creator5/1 -> BMS/1
  [timestamp] -> BMS Power Control/4(timestamp)
  [Data] -> BMS Statistic_HeatingTemperature/2(Data)
  [ID] -> BMS Power Control/1(ID)
  [Data] -> BMS Power Infor/2(Data)
  BMS Statistic_Cell Voltage Infor/1(Message) -> Bus Creator5/7  "BMS Statistic_Cell Voltage Infor"
  [ID] -> BMSWarning_Status/1(ID)
  [Data] -> BMS Cell Battery Temperature/2(Data)
  [Data] -> BMSWarning_Status/2(Data)
  [length] -> BMS Power Control/3(length)
  [ID] -> BMS Cell Voltage Infor/1(ID)
  BMSWarning_Status/1(Message) -> Bus Creator5/3  "BMSWarning_Status"
  [timestamp] -> BMS Cell Voltage Infor/4(timestamp)
  [length] -> BMS Statistic_HeatingTemperature/3(length)
  [timestamp] -> BMS_Relay Status/4(timestamp)
  [ID] -> BMS Statistic_HeatingTemperature/1(ID)
  [length] -> BMS Statistic_Cell Voltage Infor/3(length)
  [length] -> BMS_Relay Status/3(length)
  BMS Power Control/1(Message) -> Bus Creator5/4  "BMS Power Control"
  [ID] -> BMS Power Infor/1(ID)
  [length] -> BMS Cell Voltage Infor/3(length)
  [timestamp] -> BMS Power Infor/4(timestamp)
  [ID] -> BMS Statistic_Temperature of Battery/1(ID)
  BMS Cell Voltage Infor/1(Message) -> Bus Creator5/11  "BMS Cell Voltage Infor"
  [ID] -> BMS_Relay Status/1(ID)
  [length] -> BMS Power Infor/3(length)
  [Data] -> OBC_Charger Status/2(Data)
  OBC_Charger Status/1(Message) -> Bus Creator6/1  "OBC_Charger Status"
  [length] -> OBC_Charger Status/3(length)
  [ID] -> OBC_Charger Status/1(ID)
  Bus Creator6/1 -> OBC/1
  [timestamp] -> OBC_Charger Status/4(timestamp)
  BMS_Information2/1(Message) -> Bus Creator5/2  "BMS_Information2"
  BMS_Information1/1(Message) -> Bus Creator5/1  "BMS_Information1"
  [ID] -> BMS_Information2/1(ID)
  [Data] -> BMS_Information2/2(Data)
  [length] -> BMS_Information2/3(length)
  [timestamp] -> BMS_Information1/4(timestamp)
  [length] -> BMS_Information1/3(length)
  [Data] -> BMS_Information1/2(Data)
  [ID] -> BMS_Information1/1(ID)
  [timestamp] -> BMS_Information2/4(timestamp)
  [Data] -> BMS Cell HeatingTemperature/2(Data)
  BMS Cell HeatingTemperature/1(Message) -> Bus Creator5/13  "BMS Cell HeatingTemperature"
  [timestamp] -> BMS Cell HeatingTemperature/4(timestamp)
  [length] -> BMS Cell HeatingTemperature/3(length)
  [ID] -> BMS Cell HeatingTemperature/1(ID)
  [ID] -> BMS Cell Pole Temperature/1(ID)
  [length] -> BMS Cell Pole Temperature/3(length)
  [timestamp] -> BMS Cell Pole Temperature/4(timestamp)
  BMS Cell Pole Temperature/1(Message) -> Bus Creator5/14  "BMS Cell Pole Temperature"
  [Data] -> BMS Cell Pole Temperature/2(Data)
  [Data] -> BMS CumuCap Infor/2(Data)
  BMS CumuCap Infor/1(Message) -> Bus Creator5/15  "BMS CumuCap Infor"
  [timestamp] -> BMS CumuCap Infor/4(timestamp)
  [length] -> BMS CumuCap Infor/3(length)
  [ID] -> BMS CumuCap Infor/1(ID)
  [ID] -> BMS other Information1/1(ID)
  [length] -> BMS other Information1/3(length)
  [timestamp] -> BMS other Information1/4(timestamp)
  BMS other Information1/1(Message) -> Bus Creator5/16  "BMS other Information1"
  [Data] -> BMS other Information1/2(Data)
  [Data] -> "BMS other Information2 "/2(Data)
  "BMS other Information2 "/1(Message) -> Bus Creator5/17  "BMS other Information2"
  [timestamp] -> "BMS other Information2 "/4(timestamp)
  [length] -> "BMS other Information2 "/3(length)
  [ID] -> "BMS other Information2 "/1(ID)
  [ID] -> BMS_Relay Status2/1(ID)
  [length] -> BMS_Relay Status2/3(length)
  [timestamp] -> BMS_Relay Status2/4(timestamp)
  BMS_Relay Status2/1(Message) -> Bus Creator5/18  "BMS_Relay Status2"
  [Data] -> BMS_Relay Status2/2(Data)
  [Data] -> BMS_Relay Status3/2(Data)
  BMS_Relay Status3/1(Message) -> Bus Creator5/19  "BMS_Relay Status3"
  [timestamp] -> BMS_Relay Status3/4(timestamp)
  [length] -> BMS_Relay Status3/3(length)
  [ID] -> BMS_Relay Status3/1(ID)
  [ID] -> BMS Statistic_Cell ExtremumIndex Infor/1(ID)
  [length] -> BMS Statistic_Cell ExtremumIndex Infor/3(length)
  [timestamp] -> BMS Statistic_Cell ExtremumIndex Infor/4(timestamp)
  BMS Statistic_Cell ExtremumIndex Infor/1(Message) -> Bus Creator5/20  "BMS Statistic_Cell ExtremumIndex Infor"
  [Data] -> BMS Statistic_Cell ExtremumIndex Infor/2(Data)
  [Data] -> "BMS _SystemTime "/2(Data)
  "BMS _SystemTime "/1(Message) -> Bus Creator5/21  "BMS _SystemTime"
  [timestamp] -> "BMS _SystemTime "/4(timestamp)
  [length] -> "BMS _SystemTime "/3(length)
  [ID] -> "BMS _SystemTime "/1(ID)
  [ID] -> BMS CumuTimeInfor1/1(ID)
  [length] -> BMS CumuTimeInfor1/3(length)
  [timestamp] -> BMS CumuTimeInfor1/4(timestamp)
  BMS CumuTimeInfor1/1(Message) -> Bus Creator5/22  "BMS CumuTimeInfor1"
  [Data] -> BMS CumuTimeInfor1/2(Data)
  [Data] -> BMS CumuTimeInfor2/2(Data)
  BMS CumuTimeInfor2/1(Message) -> Bus Creator5/23  "BMS CumuTimeInfor2"
  [timestamp] -> BMS CumuTimeInfor2/4(timestamp)
  [length] -> BMS CumuTimeInfor2/3(length)
  [ID] -> BMS CumuTimeInfor2/1(ID)
  [ID] -> BMS other Information3/1(ID)
  [length] -> BMS other Information3/3(length)
  [timestamp] -> BMS other Information3/4(timestamp)
  BMS other Information3/1(Message) -> Bus Creator5/24  "BMS other Information3"
  [Data] -> BMS other Information3/2(Data)
  [Data] -> BMS StartDia_Infor1/2(Data)
  BMS StartDia_Infor1/1(Message) -> Bus Creator5/25  "BMS StartDia_Infor1"
  [timestamp] -> BMS StartDia_Infor1/4(timestamp)
  [length] -> BMS StartDia_Infor1/3(length)
  [ID] -> BMS StartDia_Infor1/1(ID)
  [ID] -> BMS StartDia_Infor2/1(ID)
  [length] -> BMS StartDia_Infor2/3(length)
  [timestamp] -> BMS StartDia_Infor2/4(timestamp)
  BMS StartDia_Infor2/1(Message) -> Bus Creator5/26  "BMS StartDia_Infor2"
  [Data] -> BMS StartDia_Infor2/2(Data)
  [Data] -> BMS HeatInfor/2(Data)
  BMS HeatInfor/1(Message) -> Bus Creator5/27  "BMS HeatInfor"
  [timestamp] -> BMS HeatInfor/4(timestamp)
  [length] -> BMS HeatInfor/3(length)
  [ID] -> BMS HeatInfor/1(ID)
  [timestamp] -> TMS2VCU/4(timestamp)
  Bus Creator8/1 -> TMS/1
  [ID] -> TMS2VCU/1(ID)
  [length] -> TMS2VCU/3(length)
  TMS2VCU/1(Message) -> Bus Creator8/1  "TMS2VCU"
  [Data] -> TMS2VCU/2(Data)
  [Data] -> BRS2VCU1/2(Data)
  BRS2VCU1/1(Message) -> Bus Creator9/1  "BRS2VCU1"
  [length] -> BRS2VCU1/3(length)
  [ID] -> BRS2VCU1/1(ID)
  Bus Creator9/1 -> "BRS "/1
  [timestamp] -> BRS2VCU1/4(timestamp)
  [timestamp] -> BRS2VCU2/4(timestamp)
  [ID] -> BRS2VCU2/1(ID)
  [length] -> BRS2VCU2/3(length)
  [Data] -> BRS2VCU2/2(Data)
  [Data] -> BRS2VCU3/2(Data)
  [length] -> BRS2VCU3/3(length)
  [ID] -> BRS2VCU3/1(ID)
  [timestamp] -> BRS2VCU3/4(timestamp)
  BRS2VCU2/1(Message) -> Bus Creator9/2  "BRS2VCU2"
  BRS2VCU3/1(Message) -> Bus Creator9/3  "BRS2VCU3"
  length/1 -> [length]
  ID/1 -> [ID]
  timestamp/1 -> [timestamp]
  Data/1 -> [Data]

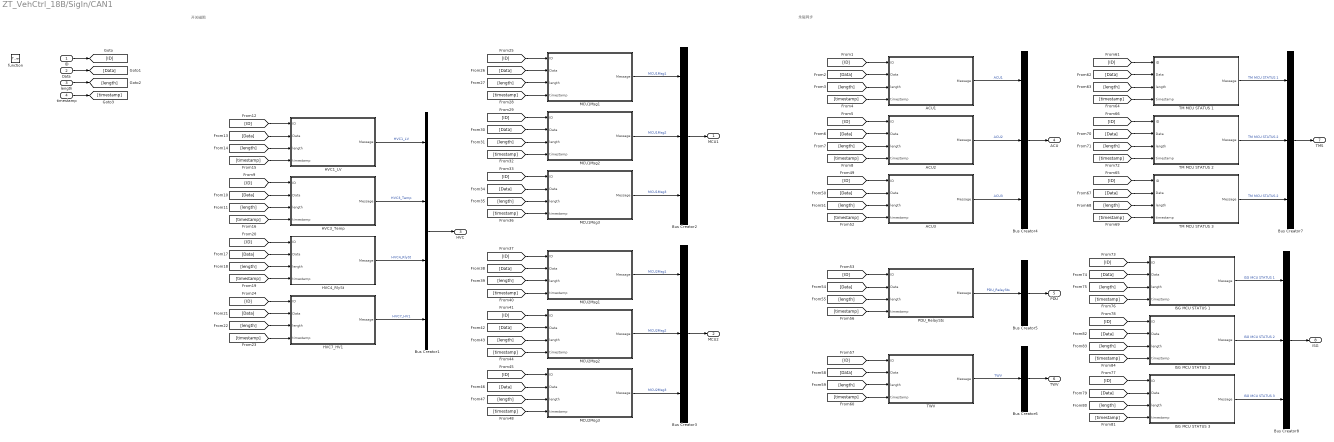
== system ZT_VehCtrl_18B/SigIn/CAN1 ==
  note: 永磁同步
  note: 开关磁阻
  ID : Inport
  Data : Inport  Port=2
  length : Inport  Port=3
  timestamp : Inport  Port=4
  function : TriggerPort  TriggerType=function-call  VariantControl=Variant
  ACU1 : Subsystem
  ACU2 : Subsystem
  ACU3 : Subsystem
  Bus Creator1 : BusCreator  Inputs=4
  Bus Creator{2..4,7..8} (5 alike) : BusCreator  Inputs=3
  Bus Creator5 : BusCreator  Inputs=1
  Bus Creator6 : BusCreator  Inputs=1
  HVC1_LV : Subsystem
  HVC3_Temp : Subsystem
  HVC4_RlySt : Subsystem
  HVC7_HV1 : Subsystem
  ISG MCU STATUS 1 : Subsystem
  ISG MCU STATUS 2 : Subsystem
  ISG MCU STATUS 3 : Subsystem
  MCU1Msg1 : Subsystem
  MCU1Msg2 : Subsystem
  MCU1Msg3 : Subsystem
  MCU2Msg1 : Subsystem
  MCU2Msg2 : Subsystem
  MCU2Msg3 : Subsystem
  PDU_RelaySts : Subsystem
  TM MCU STATUS 1 : Subsystem
  TM MCU STATUS 2 : Subsystem
  TM MCU STATUS 3 : Subsystem
  "TWV " : Subsystem
  MCU1 : Outport
  MCU2 : Outport  Port=2
  HVC : Outport  Port=3
  ACU : Outport  Port=4
  PDU : Outport  Port=5
  TWV : Outport  Port=6
  TMS : Outport  Port=7
  "ISG " : Outport  Port=8
  wires:
  length/1 -> [length]
  timestamp/1 -> [timestamp]
  Data/1 -> [Data]
  ID/1 -> [ID]
  Bus Creator2/1 -> MCU1/1
  [Data] -> HVC1_LV/2(Data)
  [timestamp] -> HVC1_LV/4(timestamp)
  [ID] -> HVC1_LV/1(ID)
  HVC1_LV/1(Message) -> Bus Creator1/1  "HVC1_LV"
  [length] -> HVC1_LV/3(length)
  [length] -> HVC3_Temp/3(length)
  HVC3_Temp/1(Message) -> Bus Creator1/2  "HVC3_Temp"
  [ID] -> HVC3_Temp/1(ID)
  [timestamp] -> HVC3_Temp/4(timestamp)
  [Data] -> HVC3_Temp/2(Data)
  [Data] -> HVC4_RlySt/2(Data)
  [timestamp] -> HVC4_RlySt/4(timestamp)
  [ID] -> HVC4_RlySt/1(ID)
  [length] -> HVC4_RlySt/3(length)
  HVC4_RlySt/1(Message) -> Bus Creator1/3  "HVC4_RlySt"
  HVC7_HV1/1(Message) -> Bus Creator1/4  "HVC7_HV1"
  [length] -> HVC7_HV1/3(length)
  [ID] -> HVC7_HV1/1(ID)
  [timestamp] -> HVC7_HV1/4(timestamp)
  [Data] -> HVC7_HV1/2(Data)
  [length] -> MCU1Msg1/3(length)
  MCU1Msg1/1(Message) -> Bus Creator2/1  "MCU1Msg1"
  [ID] -> MCU1Msg1/1(ID)
  [timestamp] -> MCU1Msg1/4(timestamp)
  [Data] -> MCU1Msg1/2(Data)
  [Data] -> MCU1Msg2/2(Data)
  [timestamp] -> MCU1Msg2/4(timestamp)
  [ID] -> MCU1Msg2/1(ID)
  MCU1Msg2/1(Message) -> Bus Creator2/2  "MCU1Msg2"
  [length] -> MCU1Msg2/3(length)
  [length] -> MCU1Msg3/3(length)
  [ID] -> MCU1Msg3/1(ID)
  [timestamp] -> MCU1Msg3/4(timestamp)
  [Data] -> MCU1Msg3/2(Data)
  MCU1Msg3/1(Message) -> Bus Creator2/3  "MCU1Msg3"
  MCU2Msg3/1(Message) -> Bus Creator3/3  "MCU2Msg3"
  [Data] -> MCU2Msg3/2(Data)
  [timestamp] -> MCU2Msg3/4(timestamp)
  [ID] -> MCU2Msg3/1(ID)
  [length] -> MCU2Msg3/3(length)
  [length] -> MCU2Msg2/3(length)
  MCU2Msg2/1(Message) -> Bus Creator3/2  "MCU2Msg2"
  [ID] -> MCU2Msg2/1(ID)
  [timestamp] -> MCU2Msg2/4(timestamp)
  [Data] -> MCU2Msg2/2(Data)
  [Data] -> MCU2Msg1/2(Data)
  [timestamp] -> MCU2Msg1/4(timestamp)
  [ID] -> MCU2Msg1/1(ID)
  MCU2Msg1/1(Message) -> Bus Creator3/1  "MCU2Msg1"
  [length] -> MCU2Msg1/3(length)
  ACU3/1(Message) -> Bus Creator4/3  "ACU3"
  [Data] -> ACU3/2(Data)
  [timestamp] -> ACU3/4(timestamp)
  [ID] -> ACU3/1(ID)
  [length] -> ACU3/3(length)
  [length] -> ACU2/3(length)
  ACU2/1(Message) -> Bus Creator4/2  "ACU2"
  [ID] -> ACU2/1(ID)
  [timestamp] -> ACU2/4(timestamp)
  [Data] -> ACU2/2(Data)
  [Data] -> ACU1/2(Data)
  [timestamp] -> ACU1/4(timestamp)
  [ID] -> ACU1/1(ID)
  ACU1/1(Message) -> Bus Creator4/1  "ACU1"
  [length] -> ACU1/3(length)
  Bus Creator4/1 -> ACU/1
  [length] -> PDU_RelaySts/3(length)
  [ID] -> PDU_RelaySts/1(ID)
  [timestamp] -> PDU_RelaySts/4(timestamp)
  [Data] -> PDU_RelaySts/2(Data)
  PDU_RelaySts/1(Message) -> Bus Creator5/1  "PDU_RelaySts"
  Bus Creator5/1 -> PDU/1
  Bus Creator6/1 -> TWV/1
  "TWV "/1(Message) -> Bus Creator6/1  "TWV"
  [Data] -> "TWV "/2(Data)
  [timestamp] -> "TWV "/4(timestamp)
  [ID] -> "TWV "/1(ID)
  [length] -> "TWV "/3(length)
  Bus Creator7/1 -> TMS/1
  [length] -> TM MCU STATUS 1/3(length)
  TM MCU STATUS 1/1(Message) -> Bus Creator7/1  "TM MCU STATUS 1"
  [ID] -> TM MCU STATUS 1/1(ID)
  [timestamp] -> TM MCU STATUS 1/4(timestamp)
  [Data] -> TM MCU STATUS 1/2(Data)
  [Data] -> TM MCU STATUS 2/2(Data)
  [timestamp] -> TM MCU STATUS 2/4(timestamp)
  [ID] -> TM MCU STATUS 2/1(ID)
  TM MCU STATUS 2/1(Message) -> Bus Creator7/2  "TM MCU STATUS 2"
  [length] -> TM MCU STATUS 2/3(length)
  [length] -> TM MCU STATUS 3/3(length)
  [ID] -> TM MCU STATUS 3/1(ID)
  [timestamp] -> TM MCU STATUS 3/4(timestamp)
  [Data] -> TM MCU STATUS 3/2(Data)
  TM MCU STATUS 3/1(Message) -> Bus Creator7/3  "TM MCU STATUS 2"
  ISG MCU STATUS 3/1(Message) -> Bus Creator8/3  "ISG MCU STATUS 3"
  [Data] -> ISG MCU STATUS 3/2(Data)
  [timestamp] -> ISG MCU STATUS 3/4(timestamp)
  [ID] -> ISG MCU STATUS 3/1(ID)
  [length] -> ISG MCU STATUS 3/3(length)
  [length] -> ISG MCU STATUS 2/3(length)
  ISG MCU STATUS 2/1(Message) -> Bus Creator8/2  "ISG MCU STATUS 2"
  [ID] -> ISG MCU STATUS 2/1(ID)
  [timestamp] -> ISG MCU STATUS 2/4(timestamp)
  [Data] -> ISG MCU STATUS 2/2(Data)
  [Data] -> ISG MCU STATUS 1/2(Data)
  [timestamp] -> ISG MCU STATUS 1/4(timestamp)
  [ID] -> ISG MCU STATUS 1/1(ID)
  ISG MCU STATUS 1/1(Message) -> Bus Creator8/1  "ISG MCU STATUS 1"
  [length] -> ISG MCU STATUS 1/3(length)
  Bus Creator8/1 -> "ISG "/1
  Bus Creator1/1 -> HVC/1
  Bus Creator3/1 -> MCU2/1

== system ZT_VehCtrl_18B/SigIn/DI ==
  note: DI PULLDOWN
  note: DI PULLUP
  Bus Creator : BusCreator  Inputs=14
  DI01 : mbd_mpc574x_ec_toolbox/GPIO Blocks/Digital_Input  gpio_pin=PTG5: [SIUL2_GPIO101 | General Purpose IO PG[5]]  pull_resistor=None
  DI02 : mbd_mpc574x_ec_toolbox/GPIO Blocks/Digital_Input  gpio_pin=PTG9: [SIUL2_GPIO105 | General Purpose IO PG[9]]  pull_resistor=None
  DI03 : mbd_mpc574x_ec_toolbox/GPIO Blocks/Digital_Input  gpio_pin=PTC11: [SIUL2_GPIO43 | General Purpose IO PC[11]]  pull_resistor=None
  DI04 : mbd_mpc574x_ec_toolbox/GPIO Blocks/Digital_Input  gpio_pin=PTA9: [SIUL2_GPIO9 | General Purpose IO PA[9]]  pull_resistor=None
  DI07 : mbd_mpc574x_ec_toolbox/GPIO Blocks/Digital_Input  gpio_pin=PTA0: [SIUL2_GPIO0 | General Purpose IO PA[0]]  pull_resistor=None
  DI08 : mbd_mpc574x_ec_toolbox/GPIO Blocks/Digital_Input  gpio_pin=PTD11: [SIUL2_GPIO59 | General Purpose IO PD[11]]  pull_resistor=None
  DI09 : mbd_mpc574x_ec_toolbox/GPIO Blocks/Digital_Input  gpio_pin=PTG6: [SIUL2_GPIO102 | General Purpose IO PG[6]]  pull_resistor=None
  DI10 : mbd_mpc574x_ec_toolbox/GPIO Blocks/Digital_Input  gpio_pin=PTG2: [SIUL2_GPIO98 | General Purpose IO PG[2]]  pull_resistor=None
  DI12 : mbd_mpc574x_ec_toolbox/GPIO Blocks/Digital_Input  gpio_pin=PTF13: [SIUL2_GPIO93 | General Purpose IO PF[13]]  pull_resistor=None
  DI13 : mbd_mpc574x_ec_toolbox/GPIO Blocks/Digital_Input  gpio_pin=PTG4: [SIUL2_GPIO100 | General Purpose IO PG[4]]  pull_resistor=None
  DI15 : mbd_mpc574x_ec_toolbox/GPIO Blocks/Digital_Input  gpio_pin=PTF12: [SIUL2_GPIO92 | General Purpose IO PF[12]]  pull_resistor=None
  DI16 : mbd_mpc574x_ec_toolbox/GPIO Blocks/Digital_Input  gpio_pin=PTG7: [SIUL2_GPIO103 | General Purpose IO PG[7]]  pull_resistor=None
  DI17 : mbd_mpc574x_ec_toolbox/GPIO Blocks/Digital_Input  gpio_pin=PTD10: [SIUL2_GPIO58 | General Purpose IO PD[10]]  pull_resistor=None
  DI18 : mbd_mpc574x_ec_toolbox/GPIO Blocks/Digital_Input  gpio_pin=PTG10: [SIUL2_GPIO106 | General Purpose IO PG[10]]  pull_resistor=None
  DI_31_32_33_34 : Subsystem  Commented=on
  Data Store Read : DataStoreRead  DataStoreName=DI07
  Data Store Read1 : DataStoreRead  DataStoreName=DI10
  Data Store Read10 : DataStoreRead  DataStoreName=DI04
  Data Store Read11 : DataStoreRead  DataStoreName=DI12
  Data Store Read12 : DataStoreRead  DataStoreName=DI08
  Data Store Read13 : DataStoreRead  DataStoreName=DI09
  Data Store Read2 : DataStoreRead  DataStoreName=DI13
  Data Store Read3 : DataStoreRead  DataStoreName=DI15
  Data Store Read4 : DataStoreRead  DataStoreName=DI16
  Data Store Read5 : DataStoreRead  DataStoreName=DI17
  Data Store Read6 : DataStoreRead  DataStoreName=DI18
  Data Store Read7 : DataStoreRead  DataStoreName=DI01
  Data Store Read8 : DataStoreRead  DataStoreName=DI02
  Data Store Read9 : DataStoreRead  DataStoreName=DI03
  Data Store Write : DataStoreWrite  DataStoreName=DI07
  Data Store Write1 : DataStoreWrite  DataStoreName=DI01
  Data Store Write10 : DataStoreWrite  DataStoreName=DI04
  Data Store Write11 : DataStoreWrite  DataStoreName=DI12
  Data Store Write12 : DataStoreWrite  DataStoreName=DI08
  Data Store Write13 : DataStoreWrite  DataStoreName=DI09
  Data Store Write2 : DataStoreWrite  DataStoreName=DI10
  Data Store Write3 : DataStoreWrite  DataStoreName=DI13
  Data Store Write4 : DataStoreWrite  DataStoreName=DI15
  Data Store Write5 : DataStoreWrite  DataStoreName=DI16
  Data Store Write6 : DataStoreWrite  DataStoreName=DI17
  Data Store Write7 : DataStoreWrite  DataStoreName=DI18
  Data Store Write8 : DataStoreWrite  DataStoreName=DI02
  Data Store Write9 : DataStoreWrite  DataStoreName=DI03
  DI : Outport
  wires:
  DI07/1 -> Data Store Write/1
  DI01/1 -> Data Store Write1/1
  DI10/1 -> Data Store Write2/1
  DI13/1 -> Data Store Write3/1
  DI15/1 -> Data Store Write4/1
  DI17/1 -> Data Store Write6/1
  DI16/1 -> Data Store Write5/1
  DI18/1 -> Data Store Write7/1
  DI09/1 -> Data Store Write13/1
  DI08/1 -> Data Store Write12/1
  DI12/1 -> Data Store Write11/1
  DI04/1 -> Data Store Write10/1
  DI02/1 -> Data Store Write8/1
  DI03/1 -> Data Store Write9/1
  Data Store Read/1 -> Bus Creator/1  "DI07"
  Data Store Read1/1 -> Bus Creator/2  "DI10"
  Data Store Read2/1 -> Bus Creator/3  "DI13"
  Data Store Read3/1 -> Bus Creator/4  "DI15"
  Data Store Read4/1 -> Bus Creator/5  "DI16"
  Data Store Read5/1 -> Bus Creator/6  "DI17"
  Data Store Read6/1 -> Bus Creator/7  "DI18"
  Data Store Read7/1 -> Bus Creator/8  "DI01"
  Data Store Read8/1 -> Bus Creator/9  "DI02"
  Data Store Read9/1 -> Bus Creator/10  "DI03"
  Data Store Read10/1 -> Bus Creator/11  "DI04"
  Data Store Read11/1 -> Bus Creator/12  "DI12"
  Data Store Read12/1 -> Bus Creator/13  "DI08"
  Data Store Read13/1 -> Bus Creator/14  "DI09"
  Bus Creator/1 -> DI/1
